simulink library "common_lib"  (R2023a)
settings: Solver=ode45  StartTime=0.0  StopTime=10.0  RelTol=1e-3
undefined symbols (not defined in the file): ACCEL_PRE_MULT, APDT_SrvcMgr_IRVHVDCSubFcnReq, C_C1GearNumbers, C_C1GearRatios, C_Calibration, C_DitherWaveform, C_GearOffset, C_GearRatioIn, C_GearRatioInverseOut, C_GearRatioOut, CLUTCH_INNER_LOOP_UPDATE_RATE, CONSTANT, DEGRADED_MODE_SIZE, Dem_EventStatusType, DiscIntNeverNeededParam, F_FAULT_ENUM, F_NOFAULT, F_OUTOFRANGE, F_RATELIMIT, FALSE, FMI14_SPECIAL_INSTRUCTIONS, FMI20_DATA_DRIFTED_HIGH, FMI21_DATA_DRIFTED_LOW, FMI29_RESERVED_FOR_SAE_ASSIGNMENT, FMI30_RESERVED_FOR_SAE_ASSIGNMENT, FMI31_CONDITION_EXISTS, FMI32_NO_FAULT, IC, k_accel, k_mean, MAX_UINT32, MEAN_PRE_MULT, NTriggers, QLTY_SIGNAL_FAILED, QLTY_SIGNAL_FULLY_FUNCTION, QLTY_SIGNAL_SUBSTITUTED_BY_1ST_CHOICE, QLTY_SIGNAL_SUBSTITUTED_BY_2ND_CHOICE, QLTY_SIGNAL_SUBSTITUTED_BY_3RD_CHOICE, QLTY_SIGNAL_SUBSTITUTED_BY_4TH_CHOICE, SAMPLE_TIME_100us, SAMPLETIME_10ms_Int, SATURATION_U16, simin, T_TestPoint, TF_FALSE, TF_TRUE, TimeStep, TRUE, WORKSPACE_UPDATE_RATE, ZERO, Zero
libraries: $bdroot x123, simulink x28, simulink_extras x4, MBD_EPS_Local_Blockset x4
(part 5 of 10)

== system common_lib/Diag/Fault Counter w Hold ==
  note: Common Library::Diagnostics::Fault Counter with Hold
  fl : Inport  OutDataTypeStr=boolean
  hold : Inport  Port=2
  true_count : Inport  Port=3
  false_count : Inport  Port=4
  fc_level : Inport  Port=5
  reset : Inport  Port=6  OutDataTypeStr=boolean
  Constant1 : Constant  Value=ZERO
  Constant2 : Constant  Value=false
  Constant3 : Constant  Value=true
  Constant4 : Constant  Value=ZERO
  Constant5 : Constant  Value=false
  Constant6 : Constant  Value=ZERO
  Logical Operator : Logic  Operator=OR
  Relay : $bdroot/Slink/Relay  init=false
      settings: AttributesFormatString=ic=%<init>
  Sat : $bdroot/Slink/Sat
  Sum : Sum  Inputs=++|  InputSameDT=on  OutDataTypeStr=Inherit: Same as first input
  Unit Delay : UnitDelay  InitialCondition=ZERO  SampleTime=-1  HasFrameUpgradeWarning=on
      settings: AttributesFormatString=ic=%<X0>
  Unit Delay1 : UnitDelay  InitialCondition=true  SampleTime=-1  HasFrameUpgradeWarning=on
      settings: AttributesFormatString=ic=%<X0>
  inc switch : Switch  Threshold=0.5  ZeroCross=off  SaturateOnIntegerOverflow=off
  inc switch1 : Switch  Threshold=0.5  ZeroCross=off  SaturateOnIntegerOverflow=off
  reset switch1 : Switch  Threshold=0.5  ZeroCross=off  SaturateOnIntegerOverflow=off
  fc : Outport  VectorParamsAs1DForOutWhenUnconnected=off
  wires:
  inc switch1/1 -> Sum/2
  Constant4/1 -> inc switch1/1
  hold/1 -> inc switch1/2
  Sum/1 -> reset switch1/3
  Constant6/1 -> reset switch1/1
  Relay/1 -> fc/1
  Constant3/1 -> Relay/4
  Constant2/1 -> Relay/5
  Constant1/1 -> Relay/3, Sat/3
  fc_level/1 -> Relay/2, Sat/2
  Sat/1 -> Unit Delay/1
  inc switch/1 -> inc switch1/3
  true_count/1 -> inc switch/1
  fl/1 -> inc switch/2
  false_count/1 -> inc switch/3
  Constant5/1 -> Unit Delay1/1
  Unit Delay1/1 -> Logical Operator/2
  reset/1 -> Logical Operator/1
  Logical Operator/1 -> reset switch1/2
  Unit Delay/1 -> Sum/1
  reset switch1/1 -> Relay/1, Sat/1

== system common_lib/Diag/Fault Injection ==
  note: Common Library::Diagnostics::Fault Injection
  input : Inport
  gain : Inport  Port=2
  offset : Inport  Port=3
  ulim : Inport  Port=4
  llim : Inport  Port=5
  hold : Inport  Port=6
  fl_trigger : Inport  Port=7
  Gain and Offset (in) : $bdroot/SCond/Gain and Offset (in)  DataType=Double
  OOR Fault Detection : $bdroot/Diag/OOR Fault Detection  InitialValue=InitialValue
  Switch : Switch  Threshold=0.5  ZeroCross=off  SaturateOnIntegerOverflow=off  InputSameDT=off
  Unit Delay : UnitDelay  InitialCondition=InitialValue  SampleTime=-1  HasFrameUpgradeWarning=on
  output : Outport  VectorParamsAs1DForOutWhenUnconnected=off
  hwfl : Outport  Port=2  VectorParamsAs1DForOutWhenUnconnected=off
  wires:
  Gain and Offset (in)/1 -> Switch/3
  Switch/1 -> OOR Fault Detection/1
  Unit Delay/1 -> Switch/1
  hold/1 -> Switch/2
  llim/1 -> OOR Fault Detection/3
  ulim/1 -> OOR Fault Detection/2
  fl_trigger/1 -> OOR Fault Detection/4
  OOR Fault Detection/2 -> hwfl/1
  OOR Fault Detection/1 -> Unit Delay/1, output/1
  offset/1 -> Gain and Offset (in)/3
  gain/1 -> Gain and Offset (in)/2
  input/1 -> Gain and Offset (in)/1

== system common_lib/Diag/Fault Log ==
  note: Common Library::Diagnostics::Fault Log
  HWfl_Active : Inport  OutDataTypeStr=boolean
  HWfl_Events : Inport  Port=2  OutDataTypeStr=uint16
  HWfl_Frames : Inport  Port=3  OutDataTypeStr=uint32
  hold : Inport  Port=4  OutDataTypeStr=boolean
  Constant1 : Constant  Value=EVENT_ZERO
  Constant18 : Constant  Value=EVENT_MAX
  Constant2 : Constant  Value=EVENT_ONE
  Constant3 : Constant  Value=FRAME_ZERO
  Constant4 : Constant  Value=FRAME_MAX
  Constant5 : Constant  Value=FRAME_ONE
  Logical Operator1 : Logic
  Logical Operator3 : Logic
  Logical Operator8 : Logic
  Sat : $bdroot/Slink/Sat
  Sat1 : $bdroot/Slink/Sat
  Sum : Sum  Inputs=|++  InputSameDT=on  OutDataTypeStr=Inherit: Same as first input
  Sum1 : Sum  Inputs=|++  InputSameDT=on  OutDataTypeStr=Inherit: Same as first input
  Unit Delay1 : UnitDelay  InitialCondition=false  SampleTime=-1  HasFrameUpgradeWarning=on
  not1 : Logic  Operator=NOT
  not2 : Logic  Operator=NOT
  reset switch : Switch  Criteria=u2 ~= 0  Threshold=0.5  ZeroCross=off  SaturateOnIntegerOverflow=off
  reset switch1 : Switch  Criteria=u2 ~= 0  Threshold=0.5  ZeroCross=off  SaturateOnIntegerOverflow=off
  events : Outport  VectorParamsAs1DForOutWhenUnconnected=off
  frames : Outport  Port=2  VectorParamsAs1DForOutWhenUnconnected=off
  wires:
  Logical Operator3/1 -> reset switch/2
  Logical Operator8/1 -> not1/1, Logical Operator3/1
  Unit Delay1/1 -> Logical Operator3/2
  not1/1 -> Unit Delay1/1
  Logical Operator1/1 -> reset switch1/2
  hold/1 -> not2/1
  not2/1 -> Logical Operator8/2, Logical Operator1/1
  HWfl_Frames/1 -> Sum1/2, reset switch1/3
  HWfl_Events/1 -> Sum/2, reset switch/3
  Constant5/1 -> Sum1/1
  Sat1/1 -> frames/1
  Sum1/1 -> reset switch1/1
  reset switch1/1 -> Sat1/1
  Constant3/1 -> Sat1/3
  Constant4/1 -> Sat1/2
  Constant2/1 -> Sum/1
  Sat/1 -> events/1
  Sum/1 -> reset switch/1
  reset switch/1 -> Sat/1
  Constant1/1 -> Sat/3
  Constant18/1 -> Sat/2
  HWfl_Active/1 -> Logical Operator1/2, Logical Operator8/1

== system common_lib/Diag/Fault_Cntr ==
  note: Common Library::Diagnostics::Fault Counter
  fl : Inport  OutDataTypeStr=boolean
  reset : Inport  Port=2  OutDataTypeStr=boolean
  fmi : Inport  Port=3  OutDataTypeStr=uint16
  Constant1 : Constant  Value=up_cnt
  Constant10 : Constant  Value=red_light  OutDataTypeStr=boolean
  Constant2 : Constant  Value=dn_cnt
  Constant3 : Constant  Value=fc_level  OutDataTypeStr=int16
  Constant4 : Constant  Value=fault_id  OutDataTypeStr=uint16
  Constant6 : Constant  Value=amber_light  OutDataTypeStr=boolean
  Data Type Conversion : DataTypeConversion  OutDataTypeStr=uint16  SaturateOnIntegerOverflow=off  RndMeth=Floor
  Data Type Conversion1 : DataTypeConversion  OutDataTypeStr=boolean  SaturateOnIntegerOverflow=off  RndMeth=Floor
  Data Type Conversion2 : DataTypeConversion  OutDataTypeStr=int16  SaturateOnIntegerOverflow=off  RndMeth=Floor
  Data Type Conversion3 : DataTypeConversion  OutDataTypeStr=int16  SaturateOnIntegerOverflow=off  RndMeth=Floor
  FaultHandlerCoreLogic : Subsystem  TreatAsAtomicUnit=on  RTWFcnName=FC_FMI_Handler
      settings: RTWFcnNameOpts=User specified  RTWFileNameOpts=Use function name
  Signal Conversion : SignalConversion  ConversionOutput=Contiguous copy  OverrideOpt=on
  Signal Conversion1 : SignalConversion  ConversionOutput=Contiguous copy  OverrideOpt=on
  inc switch : Switch  Criteria=u2 ~= 0  Threshold=0.5  ZeroCross=off  SaturateOnIntegerOverflow=off
  fc : Outport  OutDataTypeStr=uint16  VectorParamsAs1DForOutWhenUnconnected=off
  lights : Outport  Port=2  OutDataTypeStr=uint8  VectorParamsAs1DForOutWhenUnconnected=off
  wires:
  fl/1 -> inc switch/2
  reset/1 -> Data Type Conversion1/1
  FaultHandlerCoreLogic/1(fc) -> Signal Conversion/1
  fmi/1 -> Data Type Conversion/1
  FaultHandlerCoreLogic/2(lights) -> Signal Conversion1/1
  Signal Conversion/1 -> fc/1
  Signal Conversion1/1 -> lights/1
  Data Type Conversion/1 -> FaultHandlerCoreLogic/3(fmi)
  Data Type Conversion1/1 -> FaultHandlerCoreLogic/2(reset)
  Constant2/1 -> inc switch/3
  Constant3/1 -> Data Type Conversion3/1
  Constant4/1 -> FaultHandlerCoreLogic/5(fid)
  Constant10/1 -> FaultHandlerCoreLogic/6(red)
  Constant6/1 -> FaultHandlerCoreLogic/7(amber)
  Constant1/1 -> inc switch/1
  inc switch/1 -> Data Type Conversion2/1
  Data Type Conversion2/1 -> FaultHandlerCoreLogic/1(fl)
  Data Type Conversion3/1 -> FaultHandlerCoreLogic/4(fc_level)

== system common_lib/Diag/Filter w Fault Handler ==
  input : Inport
  tau : Inport  Port=2
  override_value : Inport  Port=3
  override? : Inport  Port=4
  reset? : Inport  Port=5
  default : Inport  Port=6
  ramp_time : Inport  Port=7
  fault? : Inport  Port=8
  Data Type Conversion{,1..4} (5 alike) : DataTypeConversion  OutDataTypeStr=single  SaturateOnIntegerOverflow=off  RndMeth=Floor
  Data Type Conversion5 : DataTypeConversion  OutDataTypeStr=boolean  SaturateOnIntegerOverflow=off  RndMeth=Floor
  Data Type Conversion6 : DataTypeConversion  OutDataTypeStr=boolean  SaturateOnIntegerOverflow=off  RndMeth=Floor
  Data Type Conversion7 : DataTypeConversion  OutDataTypeStr=boolean  SaturateOnIntegerOverflow=off  RndMeth=Floor
  FilterWithFaultHandlerCoreLogic : Subsystem  TreatAsAtomicUnit=on  RTWFcnName=FLTRWROFH
      settings: RTWFcnNameOpts=User specified  RTWFileNameOpts=Use function name
  Signal Conversion : SignalConversion  ConversionOutput=Contiguous copy  OverrideOpt=on
  output : Outport  VectorParamsAs1DForOutWhenUnconnected=off
  wires:
  input/1 -> Data Type Conversion/1
  tau/1 -> Data Type Conversion1/1
  override_value/1 -> Data Type Conversion2/1
  FilterWithFaultHandlerCoreLogic/1(output) -> Signal Conversion/1
  override?/1 -> Data Type Conversion7/1
  reset?/1 -> Data Type Conversion6/1
  default/1 -> Data Type Conversion3/1
  ramp_time/1 -> Data Type Conversion4/1
  fault?/1 -> Data Type Conversion5/1
  Signal Conversion/1 -> output/1
  Data Type Conversion/1 -> FilterWithFaultHandlerCoreLogic/1(input)
  Data Type Conversion1/1 -> FilterWithFaultHandlerCoreLogic/2(tau)
  Data Type Conversion2/1 -> FilterWithFaultHandlerCoreLogic/3(override_value)
  Data Type Conversion3/1 -> FilterWithFaultHandlerCoreLogic/6(default)
  Data Type Conversion4/1 -> FilterWithFaultHandlerCoreLogic/7(ramp_time)
  Data Type Conversion5/1 -> FilterWithFaultHandlerCoreLogic/8(fault?)
  Data Type Conversion6/1 -> FilterWithFaultHandlerCoreLogic/5(reset?)
  Data Type Conversion7/1 -> FilterWithFaultHandlerCoreLogic/4(override?)

== system common_lib/Diag/Filter w Fault Handler1 ==
  note: Common Library::Diagnostics::Filter With Fault Handler
  input : Inport
  tau : Inport  Port=2
  reset? : Inport  Port=3
  default : Inport  Port=4
  ramp_time : Inport  Port=5
  fault? : Inport  Port=6
  Abs1 : Abs  ZeroCross=off  SaturateOnIntegerOverflow=off
  Abs2 : Abs  ZeroCross=off  SaturateOnIntegerOverflow=off
  Constant5 : Constant  Value=TimeStep
  Fltr_wRO : Subsystem  RTWFcnName=FLTRWRO  mask(CL Filter wRO){TimeStep=TimeStep}
      mask prompts: TimeStep "Time Step"
      mask help:
      | First Order Filter, y(n)= T/tau x(n) + (1 - T/tau) y(n-1)
      |
      | If override is true (1) then output=override_value
      | If      reset is true (1) then output=input
      |    otherwise output = previous output + (input - previous output) * T/tau
      |
      | X(1) = input
      | X(2) = tau
      | X(3) = override value
      | X(4) = override flag
      | X(5) = reset flag
      |
      | Y(1) = output
      |
      | Time step is entered via mask parameter.
      | NgEK, Inc.
      mask init:
      | switch class(TimeStep)
      |  case ('double')
      |       IC = double(0.0);
      |     case ('single')
      |        IC = single(0.0);
      |     case ('int8')
      |          IC = int8(0);
      |     case ('int16')
      |       IC = int16(0);
      |    case ('int32')
      |         IC = int32(0);
      | end;
      settings: RTWFileNameOpts=Use function name
      mask Help: web(which(['common_lib17.html']))
      mask Display:
      | patch([0.4 0.4 0.6 0.6], [0.35 0.65 0.65 0.35], [255/255 127/255 255/255])
      | disp('Filter\nw RO')
      | port_label('input', 1, 'input')
      | port_label('input', 2, 'tau')
      | port_label('input', 3, 'override_value')
      | port_label('input', 4, 'override?')
      | port_label('input', 5, 'reset?')
      | port_label('output', 1, 'output')
  Product1 : Product  Inputs=**/  InputSameDT=on  OutDataTypeStr=Inherit: Same as first input
  Sum1 : Sum  Inputs=+-|  InputSameDT=on  OutDataTypeStr=Inherit: Same as first input
  Sum2 : Sum  Inputs=+-|  InputSameDT=on  OutDataTypeStr=Inherit: Same as first input
  Sum3 : Sum  Inputs=+-|  InputSameDT=on  OutDataTypeStr=Inherit: Same as first input
  Switch{1..4} (4 alike) : Switch  Threshold=0.5  ZeroCross=off  SaturateOnIntegerOverflow=off
  delay : UnitDelay  InitialCondition=Zero  SampleTime=-1  HasFrameUpgradeWarning=on
  ic: signal at fault : UnitDelay  InitialCondition=Zero  SampleTime=-1  HasFrameUpgradeWarning=on
  within zero tol of corrections : RelationalOperator  Operator=<  ZeroCross=off  InputSameDT=off
  output : Outport  VectorParamsAs1DForOutWhenUnconnected=off
  wires:
  Sum3/1 -> Abs1/1
  delay/1 -> Switch2/1
  Switch3/1 -> delay/1
  within zero tol of corrections/1 -> Switch3/2
  Abs2/1 -> within zero tol of corrections/1
  Abs1/1 -> within zero tol of corrections/2
  Sum2/1 -> Switch3/1
  Switch1/1 -> Sum3/1, Sum2/1
  Switch4/1 -> Switch1/3, Sum1/1, ic: signal at fault/1
  ic: signal at fault/1 -> Switch4/1
  Product1/1 -> Abs2/1, Sum2/2
  Constant5/1 -> Product1/2
  Sum1/1 -> Product1/1
  default/1 -> Sum3/2, Switch3/3, Sum1/2
  Fltr_wRO/1(output) -> Switch4/3, output/1
  input/1 -> Switch2/3
  Switch2/1 -> Switch1/1, Fltr_wRO/1(input)
  reset?/1 -> Fltr_wRO/3(reset?)
  tau/1 -> Fltr_wRO/2(tau)
  fault?/1 -> Switch1/2, Switch4/2, Switch2/2
  ramp_time/1 -> Product1/3

== system common_lib/Diag/OOR Fault Detection ==
  note: Common Library::Diagnostics::Out of Range Fault Detection
  in : Inport
  ulim : Inport  Port=2
  llim : Inport  Port=3
  ext_fault? : Inport  Port=4
  Logical Operator : Logic  Operator=OR  Inputs=3  AllPortsSameDT=off
  Relational Operator : RelationalOperator  Operator=<  ZeroCross=off  InputSameDT=off
  Relational Operator1 : RelationalOperator  Operator=<  ZeroCross=off  InputSameDT=off
  Sat : $bdroot/Slink/Sat
  Switch : Switch  Threshold=0.5  ZeroCross=off  SaturateOnIntegerOverflow=off  InputSameDT=off
  Unit Delay : UnitDelay  InitialCondition=InitialValue  SampleTime=-1  HasFrameUpgradeWarning=on
  out : Outport  VectorParamsAs1DForOutWhenUnconnected=off
  fault? : Outport  Port=2  VectorParamsAs1DForOutWhenUnconnected=off
  wires:
  Sat/1 -> Unit Delay/1, out/1
  Switch/1 -> Sat/1
  ext_fault?/1 -> Logical Operator/3
  llim/1 -> Sat/3, Relational Operator/2
  ulim/1 -> Relational Operator1/1, Sat/2
  in/1 -> Relational Operator1/2, Relational Operator/1, Switch/3
  Relational Operator1/1 -> Logical Operator/1
  Relational Operator/1 -> Logical Operator/2
  Logical Operator/1 -> Switch/2, fault?/1
  Unit Delay/1 -> Switch/1

== system common_lib/Diag/Rate Limit Fault Detection ==
  note: Common Library::Diagnostics::Rate Limit Fault Detection
  in : Inport
  rlim : Inport  Port=2
  ext_fault? : Inport  Port=3
  Constant1 : Constant  Value=true
  Constant2 : Constant  Value=TimeStep
  Data Type Conversion : DataTypeConversion  OutDataTypeStr=single  SaturateOnIntegerOverflow=off  RndMeth=Floor
  OOR Fault Detection : $bdroot/Diag/OOR Fault Detection  InitialValue=IC
  Product1 : Product  InputSameDT=on  OutDataTypeStr=Inherit: Same as first input
  Sum1 : Sum  Inputs=-+|  InputSameDT=on  OutDataTypeStr=Inherit: Same as first input
  Sum2 : Sum  Inputs=|++  InputSameDT=on  OutDataTypeStr=Inherit: Same as first input
  Sum3 : Sum  Inputs=++|  InputSameDT=on  OutDataTypeStr=Inherit: Same as first input
  Unit Delay : UnitDelay  InitialCondition=Zero  SampleTime=-1  HasFrameUpgradeWarning=on
      settings: AttributesFormatString=ic=%<X0>
  Unit Delay1 : UnitDelay  InitialCondition=false  SampleTime=-1  HasFrameUpgradeWarning=on
      settings: AttributesFormatString=ic=%<X0>
  Unit Delay2 : UnitDelay  InitialCondition=Zero  SampleTime=-1  HasFrameUpgradeWarning=on
      settings: AttributesFormatString=ic=%<X0>
  Unit Delay3 : UnitDelay  InitialCondition=false  SampleTime=-1  HasFrameUpgradeWarning=on
      settings: AttributesFormatString=ic=%<X0>
  inc switch : Switch  Threshold=0.5  ZeroCross=off  SaturateOnIntegerOverflow=off
  inc switch1 : Switch  Threshold=0.5  ZeroCross=off  SaturateOnIntegerOverflow=off
  out : Outport  VectorParamsAs1DForOutWhenUnconnected=off
  fault? : Outport  Port=2  VectorParamsAs1DForOutWhenUnconnected=off
  wires:
  Constant2/1 -> Data Type Conversion/1
  Data Type Conversion/1 -> Product1/1
  inc switch1/1 -> Sum2/1, Sum1/2
  Unit Delay3/1 -> inc switch1/2
  Constant1/1 -> Unit Delay3/1
  Unit Delay/1 -> inc switch1/1
  Unit Delay1/1 -> inc switch/2
  Unit Delay2/1 -> Sum3/1
  Sum3/1 -> inc switch/1
  Product1/1 -> Sum3/2, inc switch/3
  rlim/1 -> Product1/2
  inc switch/1 -> Unit Delay2/1, Sum1/1, Sum2/2
  Sum2/1 -> OOR Fault Detection/2
  Sum1/1 -> OOR Fault Detection/3
  OOR Fault Detection/2 -> Unit Delay1/1, fault?/1
  OOR Fault Detection/1 -> Unit Delay/1, out/1
  ext_fault?/1 -> OOR Fault Detection/4
  in/1 -> inc switch1/3, OOR Fault Detection/1

== system common_lib/Diagnostics/CAN OOR Fault Detection ==
  note: Common Library::Diagnostics::Out of Range Fault Detection with Enable for Enum
  in : Inport
  Enable : Inport  Port=2
  Logical Operator1 : Logic  Operator=NOT  AllPortsSameDT=off  OutDataTypeStr=boolean
  Switch : Switch  Criteria=u2 ~= 0  InputSameDT=off
  detect fault : Subsystem
  false1 : Constant  Value=FALSE  OutDataTypeStr=boolean
  out : Outport  VectorParamsAs1DForOutWhenUnconnected=off
  fault? : Outport  Port=2  VectorParamsAs1DForOutWhenUnconnected=off
  wires:
  Enable/1 -> Logical Operator1/1, detect fault/Enable
  Switch/1 -> fault?/1
  false1/1 -> Switch/1
  detect fault/1(fault set) -> Switch/3
  in/1 -> out/1, detect fault/1(In1)
  Logical Operator1/1 -> Switch/2

== system common_lib/Diagnostics/Calibration Enabled Debounce ==
  diagInput : Inport
  diagStartUpComp : Inport  Port=2
  diagMaxVal : Inport  Port=3
  diagMinVal : Inport  Port=4
  diagUpCnt : Inport  Port=5
  diagDnCnt : Inport  Port=6
  diagFaultCntThresh : Inport  Port=7
  diagPassCntThresh : Inport  Port=8
  diagDbncEnab : Inport  Port=9
  diagReset : Inport  Port=10
  diagEnable : Inport  Port=11
  diagHealEn : Inport  Port=12
  DiagFaultCounter : $bdroot/Diagnostics/DiagFaultCounter  SystemSampleTime=-1  VariantActivationTime=update diagram  Latency=0  AutoFrameSizeCalculation=off
  OR : Logic  Operator=OR  AllPortsSameDT=off  OutDataTypeStr=boolean
  Relational Operator : RelationalOperator  OutDataTypeStr=boolean  ZeroCross=off  InputSameDT=off
  Relational Operator1 : RelationalOperator  Operator=<=  OutDataTypeStr=boolean  ZeroCross=off  InputSameDT=off
  diagFaultStatus : Outport  OutputWhenDisabled=reset  InitialOutput=Dem_EventStatusType.DEM_EVENT_STATUS_INIT  VectorParamsAs1DForOutWhenUnconnected=off
  wires:
  diagHealEn/1 -> DiagFaultCounter/10
  diagPassCntThresh/1 -> DiagFaultCounter/7
  diagMaxVal/1 -> Relational Operator/2
  diagMinVal/1 -> Relational Operator1/2
  Relational Operator/1 -> OR/1
  Relational Operator1/1 -> OR/2
  diagInput/1 -> Relational Operator/1, Relational Operator1/1
  OR/1 -> DiagFaultCounter/1
  diagStartUpComp/1 -> DiagFaultCounter/2
  diagReset/1 -> DiagFaultCounter/3
  diagEnable/1 -> DiagFaultCounter/4
  diagDbncEnab/1 -> DiagFaultCounter/5
  diagFaultCntThresh/1 -> DiagFaultCounter/6
  diagUpCnt/1 -> DiagFaultCounter/8
  diagDnCnt/1 -> DiagFaultCounter/9
  DiagFaultCounter/1 -> diagFaultStatus/1

== system common_lib/Diagnostics/Calibration Enabled Debounce Boolean Input ==
  diagInput : Inport
  diagStartUpComp : Inport  Port=2
  diagUpCnt : Inport  Port=3
  diagDnCnt : Inport  Port=4
  diagFaultCntThresh : Inport  Port=5
  diagPassCntThresh : Inport  Port=6
  diagDbncEnab : Inport  Port=7
  diagReset : Inport  Port=8
  diagEnable : Inport  Port=9
  diagHealEn : Inport  Port=10
  DiagFaultCounter : $bdroot/Diagnostics/DiagFaultCounter  SystemSampleTime=-1  VariantActivationTime=update diagram  Latency=0  AutoFrameSizeCalculation=off
  diagFaultStatus : Outport  OutputWhenDisabled=reset  InitialOutput=Dem_EventStatusType.DEM_EVENT_STATUS_INIT  VectorParamsAs1DForOutWhenUnconnected=off
  wires:
  DiagFaultCounter/1 -> diagFaultStatus/1
  diagDnCnt/1 -> DiagFaultCounter/9
  diagUpCnt/1 -> DiagFaultCounter/8
  diagFaultCntThresh/1 -> DiagFaultCounter/6
  diagDbncEnab/1 -> DiagFaultCounter/5
  diagEnable/1 -> DiagFaultCounter/4
  diagReset/1 -> DiagFaultCounter/3
  diagStartUpComp/1 -> DiagFaultCounter/2
  diagInput/1 -> DiagFaultCounter/1
  diagPassCntThresh/1 -> DiagFaultCounter/7
  diagHealEn/1 -> DiagFaultCounter/10

== system common_lib/Diagnostics/Calibration Enabled MinMax OOR ==
  Input : Inport
  ULim : Inport  Port=2
  LLim : Inport  Port=3
  Cal_Enable : Inport  Port=4
  Ext_Fault : Inport  Port=5
  Enabled OOR : Subsystem  mask(Enabled OOR Subsystem){InitialValue=InitialValue, InDataType=single}
      mask prompts: InitialValue "Initial Value"; InDataType "Input Data Type"
      mask init:
      | DataType = get_param(gcb, 'InDataType');
      | Capture1 = [gcb '/OOR MinMax Capture/CL MinMax Capture'];
      | Capture2 = [gcb '/OOR MinMax Capture/CL MinMax Capture1'];
      | 
      | set_param(Capture1, 'InDataType', DataType);
      | set_param(Capture2, 'InDataType', DataType);
      mask TypeOptions InDataType: single | int16
  Switch : Switch  Threshold=0.5  ZeroCross=off  SaturateOnIntegerOverflow=off  InputSameDT=off
  Switch1 : Switch  Threshold=0.5  ZeroCross=off  SaturateOnIntegerOverflow=off  InputSameDT=off
  Out : Outport  VectorParamsAs1DForOutWhenUnconnected=off
  Max_Value : Outport  Port=2  VectorParamsAs1DForOutWhenUnconnected=off
  Min_Value : Outport  Port=3  VectorParamsAs1DForOutWhenUnconnected=off
  Fault : Outport  Port=4  VectorParamsAs1DForOutWhenUnconnected=off
  wires:
  Input/1 -> Enabled OOR/1(In), Switch/3
  ULim/1 -> Enabled OOR/2(ULim)
  LLim/1 -> Enabled OOR/3(LLim)
  Ext_Fault/1 -> Enabled OOR/4(Ext_Fault), Switch1/3
  Switch/1 -> Out/1
  Switch1/1 -> Fault/1
  Enabled OOR/1(Out) -> Switch/1
  Cal_Enable/1 -> Switch1/2, Switch/2, Enabled OOR/Enable
  Enabled OOR/2(Fault) -> Switch1/1
  Enabled OOR/3(Max) -> Max_Value/1
  Enabled OOR/4(Min) -> Min_Value/1

== system common_lib/Diagnostics/Calibration Enabled MinMax RLim ==
  Input : Inport
  Rate_Limit : Inport  Port=2
  Cal_Enable : Inport  Port=3
  Ext_Fault : Inport  Port=4
  Enabled RLim : Subsystem  mask(Enablede Rate Limit Fault Detection){IC=IC, TimeStep=TimeStep, InDataType=single}
      mask prompts: IC "Initial Condition"; TimeStep "Update Time"; InDataType "Input Data Type"
      mask init:
      | DataType = get_param(gcb, 'InDataType');
      | Capture1 = [gcb '/RLim MinMax Capture/CL MinMax Capture'];
      | Capture2 = [gcb '/RLim MinMax Capture/CL MinMax Capture1'];
      | 
      | set_param(Capture1, 'InDataType', DataType);
      | set_param(Capture2, 'InDataType', DataType);
      mask TypeOptions InDataType: single | int16
  Switch : Switch  Threshold=0.5  ZeroCross=off  SaturateOnIntegerOverflow=off  InputSameDT=off
  Switch1 : Switch  Threshold=0.5  ZeroCross=off  SaturateOnIntegerOverflow=off  InputSameDT=off
  Out : Outport  VectorParamsAs1DForOutWhenUnconnected=off
  Max Pos Rate : Outport  Port=2  VectorParamsAs1DForOutWhenUnconnected=off
  Max Neg Rate : Outport  Port=3  VectorParamsAs1DForOutWhenUnconnected=off
  Fault : Outport  Port=4  VectorParamsAs1DForOutWhenUnconnected=off
  wires:
  Cal_Enable/1 -> Switch/2, Switch1/2, Enabled RLim/Enable
  Input/1 -> Switch/3, Enabled RLim/1(In)
  Switch/1 -> Out/1
  Switch1/1 -> Fault/1
  Rate_Limit/1 -> Enabled RLim/2(RLim)
  Enabled RLim/1(out) -> Switch/1
  Enabled RLim/2(fault?) -> Switch1/1
  Ext_Fault/1 -> Enabled RLim/3(Ext_Fault), Switch1/3
  Enabled RLim/3(Max Pos Rate) -> Max Pos Rate/1
  Enabled RLim/4(Max Neg Rate) -> Max Neg Rate/1

== system common_lib/Diagnostics/Ccaller_DiagLv1 ==
  diagFaultActive : Inport
  diagStartUpComp : Inport  Port=2
  diagReset : Inport  Port=3
  diagEnable : Inport  Port=4
  diagDbncEnable : Inport  Port=5
  diagFaultCntThresh : Inport  Port=6
  diagPassCntThresh : Inport  Port=7
  diagUpCnt : Inport  Port=8
  diagDnCnt : Inport  Port=9
  diagHealEn : Inport  Port=10
  diagPrestorageEn : Inport  Port=11
  diagJumpDownEn : Inport  Port=12
  DiagDebounceLv1_CCaller : CCaller  FunctionName=DiagDebounceLv1  PortSpecificationStruct="%)30     .    \\!H   8    (     @         %    \"    !$    !     0         %  0 \"0    $    V    07)G3F%M90  4&]R=$YA;64 4V-O<&4     26YD97@     5'EP90      4VEZ90         .    0     8    (    !          %    \"     $    0     0         0    $    &1I86=&875L=$-O=6YT97(.    0     8    (    !          %    \"     $    0     0         0    $    &1I86=&875L=$-O=6YT97(.    0     8    (    !          %  ...(+8912 chars)"
  Unit Delay : UnitDelay  InitialCondition=int16(0)  SampleTime=-1  HasFrameUpgradeWarning=on
      settings: AttributesFormatString=%<InitialCondition>
  Unit Delay1 : UnitDelay  InitialCondition=uint8(32)  SampleTime=-1  HasFrameUpgradeWarning=on
      settings: AttributesFormatString=%<InitialCondition>
  Unit Delay2 : UnitDelay  InitialCondition=false  SampleTime=-1  HasFrameUpgradeWarning=on
      settings: AttributesFormatString=%<InitialCondition>
  Unit Delay3 : UnitDelay  InitialCondition=false  SampleTime=-1  HasFrameUpgradeWarning=on
      settings: AttributesFormatString=%<InitialCondition>
  Unit Delay4 : UnitDelay  InitialCondition=false  SampleTime=-1  HasFrameUpgradeWarning=on
      settings: AttributesFormatString=%<InitialCondition>
  diagFaultStatus : Outport  VectorParamsAs1DForOutWhenUnconnected=off
  diagPrestorageTrigger : Outport  Port=2  VectorParamsAs1DForOutWhenUnconnected=off
  wires:
  diagJumpDownEn/1 -> DiagDebounceLv1_CCaller/17
  Unit Delay4/1 -> DiagDebounceLv1_CCaller/4
  DiagDebounceLv1_CCaller/4 -> Unit Delay4/1
  diagPrestorageEn/1 -> DiagDebounceLv1_CCaller/16
  Unit Delay3/1 -> DiagDebounceLv1_CCaller/5
  DiagDebounceLv1_CCaller/5 -> diagPrestorageTrigger/1, Unit Delay3/1
  Unit Delay2/1 -> DiagDebounceLv1_CCaller/3
  DiagDebounceLv1_CCaller/3 -> Unit Delay2/1
  Unit Delay1/1 -> DiagDebounceLv1_CCaller/2
  DiagDebounceLv1_CCaller/2 -> Unit Delay1/1, diagFaultStatus/1
  Unit Delay/1 -> DiagDebounceLv1_CCaller/1
  DiagDebounceLv1_CCaller/1 -> Unit Delay/1
  diagPassCntThresh/1 -> DiagDebounceLv1_CCaller/12
  diagDbncEnable/1 -> DiagDebounceLv1_CCaller/10
  diagEnable/1 -> DiagDebounceLv1_CCaller/9
  diagHealEn/1 -> DiagDebounceLv1_CCaller/15
  diagFaultActive/1 -> DiagDebounceLv1_CCaller/6
  diagFaultCntThresh/1 -> DiagDebounceLv1_CCaller/11
  diagReset/1 -> DiagDebounceLv1_CCaller/8
  diagDnCnt/1 -> DiagDebounceLv1_CCaller/14
  diagStartUpComp/1 -> DiagDebounceLv1_CCaller/7
  diagUpCnt/1 -> DiagDebounceLv1_CCaller/13

== system common_lib/Diagnostics/Ccaller_DiagLv2 ==
  diagFaultActive : Inport
  diagStartUpComp : Inport  Port=2
  diagReset : Inport  Port=3
  diagFaultCntThresh : Inport  Port=4
  diagUpCnt : Inport  Port=5
  diagDnCnt : Inport  Port=6
  diagHealEn : Inport  Port=7
  DiagDebounceLv2_CCaller : CCaller  FunctionName=DiagDebounceLv2  PortSpecificationStruct="%)30     .    8!$   8    (     @         %    \"     L    !     0         %  0 \"0    $    V    07)G3F%M90  4&]R=$YA;64 4V-O<&4     26YD97@     5'EP90      4VEZ90         .    ,     8    (    !          %    \"     $    #     0         0  , ;W5T  X    P    !@    @    $          4    (     0    ,    !         !   P!O=70 #@   #@    &    \"     0         !0    @    !    !@    $         $     8   !/=7 ...(+5614 chars)"
  Unit Delay : UnitDelay  InitialCondition=int16(0)  SampleTime=-1  HasFrameUpgradeWarning=on
      settings: AttributesFormatString=%<InitialCondition>
  Unit Delay1 : UnitDelay  InitialCondition=uint8(0)  SampleTime=-1  HasFrameUpgradeWarning=on
      settings: AttributesFormatString=%<InitialCondition>
  Unit Delay2 : UnitDelay  InitialCondition=int16(0)  SampleTime=-1  HasFrameUpgradeWarning=on
      settings: AttributesFormatString=%<InitialCondition>
  diagFaultStatus : Outport  VectorParamsAs1DForOutWhenUnconnected=off
  wires:
  diagUpCnt/1 -> DiagDebounceLv2_CCaller/8
  diagStartUpComp/1 -> DiagDebounceLv2_CCaller/5
  diagDnCnt/1 -> DiagDebounceLv2_CCaller/9
  diagReset/1 -> DiagDebounceLv2_CCaller/6
  DiagDebounceLv2_CCaller/1 -> diagFaultStatus/1
  diagFaultCntThresh/1 -> DiagDebounceLv2_CCaller/7
  diagFaultActive/1 -> DiagDebounceLv2_CCaller/4
  diagHealEn/1 -> DiagDebounceLv2_CCaller/10
  DiagDebounceLv2_CCaller/2 -> Unit Delay/1
  Unit Delay/1 -> DiagDebounceLv2_CCaller/1
  DiagDebounceLv2_CCaller/3 -> Unit Delay1/1
  Unit Delay1/1 -> DiagDebounceLv2_CCaller/2
  DiagDebounceLv2_CCaller/4 -> Unit Delay2/1
  Unit Delay2/1 -> DiagDebounceLv2_CCaller/3

== system common_lib/Diagnostics/DiagDbncCntr ==
  SetTime : Inport
  HealTime : Inport  Port=2
  FaultFlg : Inport  Port=3
  ResetFlg : Inport  Port=4
  Bitwise Operator4 : simulink/Logic and Bit Operations/Bitwise Operator  logicop=NOT  UseBitMask=off  BitMask=bin2dec('11011001')  BitMaskRealWorld=Stored Integer
  Counter1 : Subsystem  mask(CL Counter){IC=uint16(0)}
      mask prompts: IC "Initial condition"
      mask help:
      | Generic counter block.
      | Counts up by up_val when count_up? is true
      | Counts down by down_val when count_down? is true.
      | Block can be used as a timer if increment value is set to the frame rate.
      |
      | X(1) = increment value
      | X(2) = count up flag
      | X(3) = decrement value
      | X(4) = count down flag
      | X(5) = max counter value
      | X(6) = min counter value
      | X(7) = reset
      |
      | Y(1) = output
      |
      | Initial condition is entered via mask.
      | NgEK, Inc.
      mask init: same as common_lib/Misc/Counter
      mask Help: web(which(['common_lib23.html']))
      mask Display:
      | patch([0.4 0.4 0.6 0.6], [0.4 0.6 0.6 0.4], [255/255 127/255 255/255])
      | disp('Counter')
      | port_label('input', 1, 'up_val')
      | port_label('input', 2, 'count_up?')
      | port_label('input', 3, 'down_val')
      | port_label('input', 4, 'count_down?')
      | port_label('input', 5, 'max_count')
      | port_label('input', 6, 'min_count')
      | port_label('input', 7, 'reset?')
      | port_label('output', 1, 'output')
  Divide1 : Product  Inputs=*/  OutDataTypeStr=uint16
  Divide2 : Product  Inputs=*/  OutDataTypeStr=uint16
  Product1 : Product  OutDataTypeStr=uint32
  Product2 : Product  OutDataTypeStr=uint32
  Relay : $bdroot/Slink/Relay  init=false
  Saturation : Constant  Value=SATURATION_U16  SampleTime=-1
  Saturation1 : Constant  Value=SATURATION_U16  SampleTime=-1
  Saturation2 : Constant  Value=SATURATION_U16  SampleTime=-1
  Saturation3 : Constant  Value=0  OutDataTypeStr=uint16  SampleTime=-1
  Saturation4 : Constant  Value=TRUE  SampleTime=-1
  Saturation5 : Constant  Value=FALSE  SampleTime=-1
  TimeStep : Constant  Value=SAMPLETIME_10ms_Int  SampleTime=-1
  TimeStep1 : Constant  Value=SAMPLETIME_10ms_Int  SampleTime=-1
  FaultOut : Outport  VectorParamsAs1DForOutWhenUnconnected=off
  wires:
  HealTime/1 -> Divide2/2
  Saturation4/1 -> Relay/4
  Saturation3/1 -> Relay/3, Counter1/6(min_count)
  Divide2/1 -> Counter1/3(down_val)
  Divide1/1 -> Counter1/1(up_val)
  TimeStep/1 -> Product1/1
  Product1/1 -> Divide1/1
  Saturation2/1 -> Relay/2, Counter1/5(max_count)
  Saturation5/1 -> Relay/5
  FaultFlg/1 -> Counter1/2(count_up?), Bitwise Operator4/1
  Counter1/1(output) -> Relay/1
  TimeStep1/1 -> Product2/1
  Saturation1/1 -> Product2/2
  ResetFlg/1 -> Counter1/7(reset?)
  Saturation/1 -> Product1/2
  SetTime/1 -> Divide1/2
  Relay/1 -> FaultOut/1
  Product2/1 -> Divide2/1
  Bitwise Operator4/1 -> Counter1/4(count_down?)
